simulink library "Online_Application_Department"  (R2019a)
settings: Solver=VariableStepAuto  StartTime=0.0  StopTime=10.0  RelTol=1e-3
undefined symbols (not defined in the file or in its folder): m, n
settings Model: Creator=arsineh  LastModifiedBy=arsineh

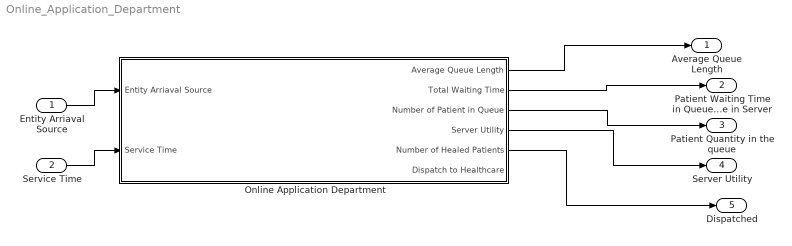
== system Online_Application_Department ==
  Entity Arriaval Source : Inport
  Service Time : Inport  Port=2
  Online Application Department : Subsystem
  Average Queue Length : Outport
  "Patient Waiting Time in Queue + Patient Examination Time in Server " : Outport  Port=2
  Patient Quantity in the queue : Outport  Port=3
  Server Utility : Outport  Port=4
  Dispatched : Outport  Port=5
  wires:
  Entity Arriaval Source/1 -> Online Application Department/1(Entity Arriaval Source)
  Online Application Department/3(Number of Patient in Queue) -> Patient Quantity in the queue/1
  Service Time/1 -> Online Application Department/2(Service Time)
  Online Application Department/1(Average Queue Length) -> Average Queue Length/1
  Online Application Department/2(Total Waiting Time) -> "Patient Waiting Time in Queue + Patient Examination Time in Server "/1
  Online Application Department/4(Server Utility) -> Server Utility/1
  Online Application Department/5(Number of Healed Patients) -> Dispatched/1

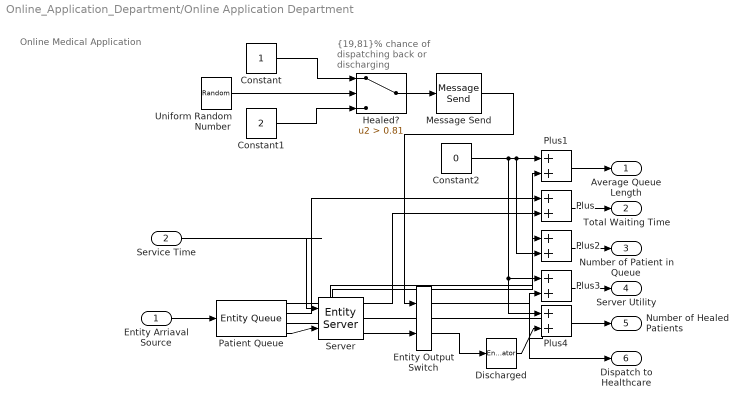
== system Online_Application_Department/Online Application Department ==
  note: Online Medical Application
  note: {19,81}% chance of
      | dispatching back or
      | discharging
  Entity Arriaval Source : Inport
  Service Time : Inport  Port=2
  Constant : Constant  VectorParams1D=off
  Constant1 : Constant  Value=2  VectorParams1D=off
  Constant2 : Constant  Value=0
  Discharged : EntityTerminator  InputPortMessageModes=m  NumberEntitiesArrived=on
      settings: OutputPortMap=o0
  Entity Output Switch : EntityOutputSwitch  InputPortMessageModes=m,m  OutputPortMessageModes=m,m  SwitchingCriterion=From control port  SwitchAttributeName=Attribute1
      settings: InputPortMap=u0,u1
  Healed? : Switch  Criteria=u2 > Threshold  Threshold=0.81
  Message Send : MessageSend  OutputPortMessageModes=m
      settings: InputPortMap=u1
  Patient Queue : EntityQueue  InputPortMessageModes=m  OutputPortMessageModes=n,n,n,m  Capacity=100000  NumberEntitiesInBlock=on  AverageWait=on  AverageQueueLength=on
      settings: OutputPortMap=o1,o2,o3,o5
  Plus{,1..4} (5 alike) : Sum
  Server : EntityServer  InputPortMessageModes=n,m  OutputPortMessageModes=n,n,m  Capacity=40  ServiceTimeSource=Signal port  AverageWait=on  Utilization=on
      settings: InputPortMap=u0,u2  OutputPortMap=o4,o5,o9
  Uniform Random Number : UniformRandomNumber  Minimum=0  Seed=1325435  SampleTime=0.1
  Average Queue Length : Outport
  Total Waiting Time : Outport  Port=2
  Number of Patient in Queue : Outport  Port=3
  Server Utility : Outport  Port=4
  Number of Healed Patients : Outport  Port=5
  Dispatch to Healthcare : Outport  Port=6
  wires:
  Uniform Random Number/1 -> Healed?/2
  Patient Queue/4 -> Server/2
  Constant1/1 -> Healed?/3
  Entity Arriaval Source/1 -> Patient Queue/1
  Patient Queue/1 -> Plus2/1
  Server/3 -> Entity Output Switch/2
  Constant/1 -> Healed?/1
  Service Time/1 -> Server/1
  Patient Queue/3 -> Plus1/2
  Healed?/1 -> Message Send/1
  Message Send/1 -> Entity Output Switch/1
  Plus/1 -> Total Waiting Time/1
  Patient Queue/2 -> Plus/1
  Server/1 -> Plus/2
  Server/2 -> Plus3/2
  Entity Output Switch/2 -> Discharged/1
  Entity Output Switch/1 -> Dispatch to Healthcare/1
  Plus1/1 -> Average Queue Length/1
  Constant2/1 -> Plus4/1, Plus3/1, Plus2/2, Plus1/1
  Plus2/1 -> Number of Patient in Queue/1
  Plus3/1 -> Server Utility/1
  Discharged/1 -> Plus4/2
  Plus4/1 -> Number of Healed Patients/1
